simulink model "OpenLoopHW"  (R2023a)
settings: Solver=FixedStepDiscrete  StartTime=0.0  StopTime=10  FixedStep=0.001  RelTol=1e-3  EnableMultiTasking=on
values from neighbouring files (symbols this model uses):
  t_control = t    [MAIN.m]    (also in MAIN_HW.m; step.mat = [0 0.10101010101 0.20202020202 0.30303030303 0.40404040404 0)
  ut = u    [MAIN.m]    (also in MAIN_HW.m; step.mat = [0 0 0 0 0 0 0 0 0 0 0.6 0.6 ... (100 elements, 1x100)])
  x0 = [-pi/2;0;0;0]    [MAIN.m]    (also in MAIN_HW.m; fitParams.m = [-pi/2; 0; 0; 0])
undefined symbols (not defined in the file or in its folder): DiscIntNeverNeededParam, HIL
libraries: quarc_library x3, simulink x2
settings Model: SimulationMode=external  ExtModeTrigType=signal  ExtModeTrigDuration=10000  ExtModeTrigDirection=either  ExtModeTrigLevel=0.500000  Creator=colegiusto  LastModifiedBy=colegiusto
settings SolverCC: PositivePriorityOrder=on
settings RTWCC: Description=QUARC Win64 Target Using Toolchain  SystemTargetFile=quarc_win64.tlc  Toolchain=QUARC win64 | nmake (64-bit Windows)  BuildConfiguration=Faster Runs
settings STFCustomTargetCC: TargetLangStandard=C89/C90 (ANSI)  SystemTargetFile=quarc_win64.tlc
settings GRTTargetCC: TargetLangStandard=C89/C90 (ANSI)  ParMdlRefBuildCompliant=off  CompOptLevelCompliant=off  CombineOutputUpdateFcns=off  MatFileLogging=off  CPPClassGenCompliant=off  GRTInterface=on  ExtMode=on  ExtModeMexFile=quarc_comm

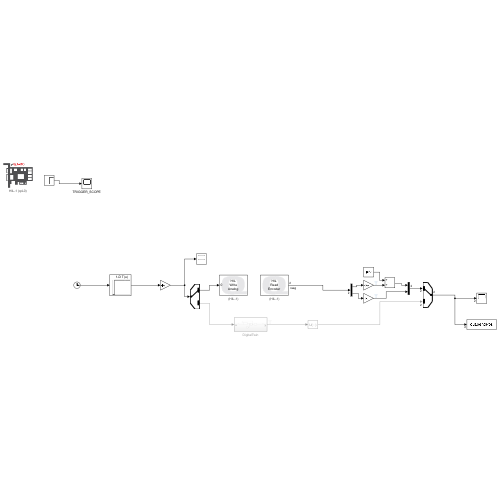
[thumbnail: Simulink's stored preview of the top-level diagram]
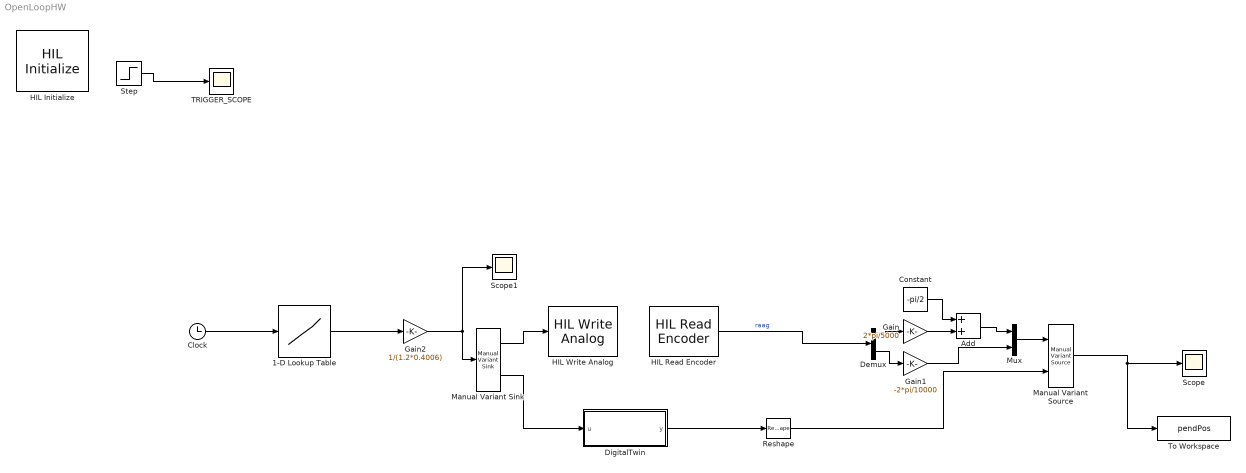
== system OpenLoopHW ==
  1-D Lookup Table : Lookup_n-D  NumberOfTableDimensions=1  BreakpointsForDimension1=t_control  Table=ut  InternalRulePriority=Speed  RndMeth=Simplest
  Add : Sum
  Clock : Clock
  Constant : Constant  Value=-pi/2
  Demux : Demux  Outputs=2
  DigitalTwin : Subsystem
  Gain : Gain  Gain=2*pi/5000
  Gain1 : Gain  Gain=-2*pi/10000
  Gain2 : Gain  Gain=1/(1.2*0.4006)
  HIL Initialize : quarc_library/Data Acquisition/Generic/Configuration/HIL Initialize  object_name=HIL-1  board_type=q4  board_number=0  board_options=""  exclusive=off  active=on  hardware_clocks=[0:1]  clock_modes=[0 0]  initial_clock_frequencies=[]  set_clock_params_at_start=on  set_clock_params_at_switch_in=off  set_clock_frequencies_at_start=off  set_clock_frequencies_at_switch_in=off  analog_input_channels=[0:3]  analog_input_configurations=[]  analog_input_maximums=10  analog_input_minimums=-10  set_analog_input_params_at_start=off  set_analog_input_params_at_switch_in=off  analog_output_channels=[0:3]  analog_output_maximums=[10]  analog_output_minimums=[-10]  initial_analog_outputs=[0]  final_analog_outputs=[0]  watchdog_analog_outputs=0  set_analog_output_params_at_start=on  set_analog_output_params_at_switch_in=off  set_analog_outputs_at_start=on  set_analog_outputs_at_switch_in=off  set_analog_outputs_at_terminate=on  set_analog_outputs_at_switch_out=off  set_analog_outputs_on_watchdog=off  digital_input_channels=[]  digital_output_channels=[]  digital_output_configuration=[]  initial_digital_outputs=[1]  final_digital_outputs=[1]  watchdog_digital_outputs=[2]  set_digital_output_params_at_start=off  set_digital_output_params_at_switch_in=off  set_digital_outputs_at_start=on  set_digital_outputs_at_switch_in=off  set_digital_outputs_at_terminate=on  set_digital_outputs_at_switch_out=off  set_digital_outputs_on_watchdog=off  encoder_channels=[0:3]  quadrature=[4]  encoder_filter_frequency=(1/60e-9)/1  initial_encoder_counts=[0]  set_encoder_params_at_start=on  set_encoder_params_at_switch_in=off  set_encoder_counts_at_start=on  set_encoder_counts_at_switch_in=off  pwm_channels=[]  pwm_modes=[0]  pwm_frequency=(1/60e-9)/1024  pwm_configuration=[]  pwm_alignment=[]  pwm_polarity=[]  pwm_leading_deadband=[]  pwm_trailing_deadband=[]  initial_pwm_outputs=[0]  final_pwm_outputs=[0]  watchdog_pwm_outputs=[]  set_pwm_params_at_start=on  set_pwm_params_at_switch_in=off  set_pwm_outputs_at_start=on  set_pwm_outputs_at_switch_in=off  set_pwm_outputs_at_terminate=on  set_pwm_outputs_at_switch_out=off  set_pwm_outputs_on_watchdog=off  other_output_channels=[]  initial_other_outputs=[]  final_other_outputs=[]  watchdog_other_outputs=[]  set_other_outputs_at_start=off  set_other_outputs_at_switch_in=off  set_other_outputs_at_terminate=off  set_other_outputs_at_switch_out=off  set_other_outputs_on_watchdog=off
  HIL Read Encoder : quarc_library/Data Acquisition/Generic/Immediate I//O/HIL Read Encoder  object_name=HIL-1  channels=[0:1]  sample_time=0.001  active=on  vector_output=on  data_type_mode=Inherit via back propagation  data_type=double
  HIL Write Analog : quarc_library/Data Acquisition/Generic/Immediate I//O/HIL Write Analog  object_name=HIL-1  channels=0  sample_time=0.001  active=off  vector_input=off
  Manual Variant Sink : simulink/Signal Routing/Manual Variant Sink  NumChoices=2  LabelModeActiveChoice=V_1
  Manual Variant Source : simulink/Signal Routing/Manual Variant Source  NumChoices=2  LabelModeActiveChoice=V_1
  Mux : Mux  Inputs=2
  Reshape : Reshape
  Scope : Scope
  Scope1 : Scope
  Step : Step  Time=0.001  SampleTime=0
  TRIGGER_SCOPE : Scope
  To Workspace : ToWorkspace  VariableName=pendPos  SaveFormat=Structure With Time  SampleTime=-1
  wires:
  HIL Read Encoder/1 -> Demux/1  "raag"
  Step/1 -> TRIGGER_SCOPE/1
  1-D Lookup Table/1 -> Gain2/1
  Demux/2 -> Gain1/1
  Demux/1 -> Gain/1
  Gain1/1 -> Mux/2
  Gain2/1 -> Manual Variant Sink/1, Scope1/1
  Clock/1 -> 1-D Lookup Table/1
  Add/1 -> Mux/1
  Gain/1 -> Add/2
  Constant/1 -> Add/1
  DigitalTwin/1(y) -> Reshape/1
  Manual Variant Sink/1 -> HIL Write Analog/1
  Manual Variant Sink/2 -> DigitalTwin/1(u)
  Mux/1 -> Manual Variant Source/1
  Manual Variant Source/1 -> To Workspace/1, Scope/1
  Reshape/1 -> Manual Variant Source/2

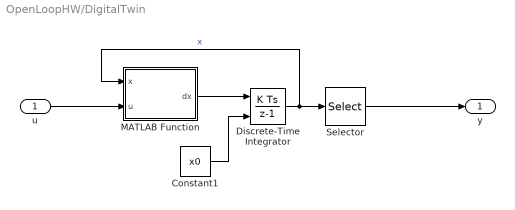
== system OpenLoopHW/DigitalTwin ==
  u : Inport
  Constant1 : Constant  Value=x0  VectorParams1D=off
  Discrete-Time Integrator : DiscreteIntegrator  InitialConditionSource=external  SampleTime=-1  ICPrevOutput=DiscIntNeverNeededParam  ICPrevScaledInput=DiscIntNeverNeededParam
  MATLAB Function : MATLAB Function  TreatAsAtomicUnit=on
  Selector : Selector  InputPortWidth=4  IndexOptions=Index vector (dialog)  Indices=[1 2]  OutputSizes=1
  y : Outport
  wires:
  Discrete-Time Integrator/1 -> Selector/1, MATLAB Function/1(x)  "x"
  Constant1/1 -> Discrete-Time Integrator/2
  MATLAB Function/1(dx) -> Discrete-Time Integrator/1
  u/1 -> MATLAB Function/2(u)
  Selector/1 -> y/1

== matlab function OpenLoopHW/DigitalTwin/MATLAB Function ==
  data: x input; u input; dx output; p parameter
function dx = dyn(x,u,p)
    dx = dynamics(x,u,p);
end
